simulink model "PIDsystem"  (Simulink 8.9)
settings: Solver=VariableStepAuto  StartTime=0.0  StopTime=10.0  RelTol=1e-3
values from neighbouring files (symbols this model uses):
  C_dirden = cell2mat(C_dirden)    [PIDsetup.m]
  C_dirnum = cell2mat(C_dirnum)    [PIDsetup.m]
  C_esqden = cell2mat(C_esqden)    [PIDsetup.m]
  C_esqnum = cell2mat(C_esqnum)    [PIDsetup.m]
  G_dirden = cell2mat(G_dirden)    [PIDsetup.m]
  G_dirnum = cell2mat(G_dirnum)    [PIDsetup.m]
  G_esqden = cell2mat(G_esqden)    [PIDsetup.m]
  G_esqnum = cell2mat(G_esqnum)    [PIDsetup.m]
  left_deadzone = pos_limit    (= 0)    [analyze_data.m]    (also in deadzone_values.mat = 1.9292; full_system.mat = 1.8942)
  right_deadzone = pos_limit    (= 0)    [analyze_data.m]    (also in deadzone_values.mat = 1.9558; full_system.mat = 1.85173333333)
  T = 0.2    [full_system.mat]    (also in get_controller.m)
settings Model: SuppressorTable=22 serialization::archive 11 0 6 0 0 0 11 0  Creator=rafael  LastModifiedBy=rafael
settings DataIOCC: LimitDataPoints=off  SaveFormat=Dataset  SignalLoggingSaveFormat=Dataset
settings OptimizationCC: LifeSpan=auto
settings DebuggingCC: UnderspecifiedInitializationDetection=Simplified  MergeDetectMultiDrivingBlocksExec=error  FcnCallInpInsideContextMsg=error  StateNameClashWarn=none  SFUnexpectedBacktrackingDiag=error  SFNoUnconditionalDefaultTransitionDiag=error  SFExecutionAtInitializationDiag=warning
settings HardwareCC: ProdBitPerPointer=64  ProdBitPerSizeT=64  ProdBitPerPtrDiffT=64  ProdLargestAtomicFloat=Float  ProdIntDivRoundTo=Zero  ProdEndianess=LittleEndian  ProdWordSize=64  ProdHWDeviceType=Intel->x86-64 (Windows64)
settings ModelReferenceCC: PropagateSignalLabelsOutOfModel=on
settings GRTTargetCC: TargetLangStandard=C99 (ISO)  GeneratePreprocessorConditionals=Use local settings  CombineOutputUpdateFcns=on  GRTInterface=off
settings ConfigComp: CovMetricSettings=dwe  CovHtmlReporting=off  CovSaveCumulativeToWorkspaceVar=off  CovSaveSingleToWorkspaceVar=off  CovExternalEMLEnable=on

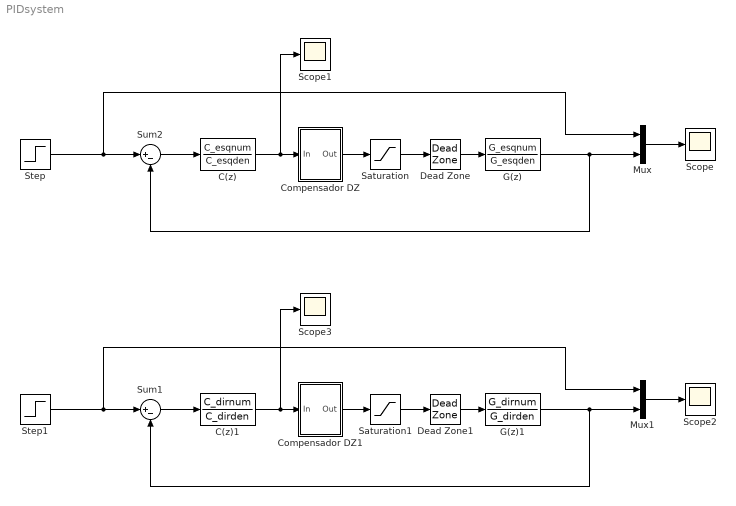
== system PIDsystem ==
  C(z) : DiscreteTransferFcn  Numerator=C_esqnum  Denominator=C_esqden
  C(z)1 : DiscreteTransferFcn  Numerator=C_dirnum  Denominator=C_dirden
  Compensador DZ : Subsystem
  Compensador DZ1 : Subsystem
  Dead Zone : DeadZone  LowerValue=-left_deadzone  UpperValue=left_deadzone  SaturateOnIntegerOverflow=on
  Dead Zone1 : DeadZone  LowerValue=-right_deadzone  UpperValue=right_deadzone  SaturateOnIntegerOverflow=on
  G(z) : DiscreteTransferFcn  Numerator=G_esqnum  Denominator=G_esqden
  G(z)1 : DiscreteTransferFcn  Numerator=G_dirnum  Denominator=G_dirden
  Mux : Mux  Inputs=2
  Mux1 : Mux  Inputs=2
  Saturation : Saturate  UpperLimit=7  LowerLimit=-7
  Saturation1 : Saturate  UpperLimit=7  LowerLimit=-7
  Scope{,1..3} (4 alike) : Scope
  Step : Step  After=3  SampleTime=T
  Step1 : Step  After=3  SampleTime=T
  Sum1 : Sum  Inputs=|+-
  Sum2 : Sum  Inputs=|+-
  wires:
  Step/1 -> Mux/1, Sum2/1
  Sum2/1 -> C(z)/1
  Compensador DZ/1(Out) -> Saturation/1
  C(z)/1 -> Scope1/1, Compensador DZ/1(In)
  Saturation/1 -> Dead Zone/1
  Dead Zone/1 -> G(z)/1
  G(z)/1 -> Mux/2, Sum2/2
  Mux/1 -> Scope/1
  Saturation1/1 -> Dead Zone1/1
  Compensador DZ1/1(Out) -> Saturation1/1
  C(z)1/1 -> Scope3/1, Compensador DZ1/1(In)
  Sum1/1 -> C(z)1/1
  Step1/1 -> Mux1/1, Sum1/1
  Dead Zone1/1 -> G(z)1/1
  G(z)1/1 -> Mux1/2, Sum1/2
  Mux1/1 -> Scope2/1

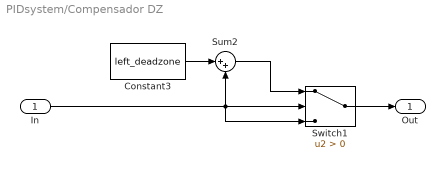
== system PIDsystem/Compensador DZ ==
  In : Inport
  Constant3 : Constant  Value=left_deadzone  SampleTime=-1
  Sum2 : Sum  Inputs=|++
  Switch1 : Switch  Criteria=u2 > Threshold
  Out : Outport
  wires:
  Switch1/1 -> Out/1
  In/1 -> Switch1/3, Switch1/2, Sum2/2
  Sum2/1 -> Switch1/1
  Constant3/1 -> Sum2/1

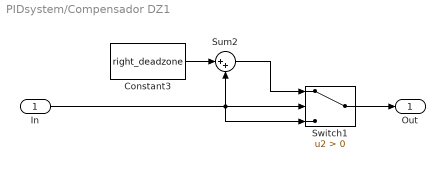
== system PIDsystem/Compensador DZ1 ==
  In : Inport
  Constant3 : Constant  Value=right_deadzone  SampleTime=-1
  Sum2 : Sum  Inputs=|++
  Switch1 : Switch  Criteria=u2 > Threshold
  Out : Outport
  wires:
  Switch1/1 -> Out/1
  In/1 -> Switch1/3, Switch1/2, Sum2/2
  Sum2/1 -> Switch1/1
  Constant3/1 -> Sum2/1
